simulink model "DigitalTwin_AI"  (R2024b)
settings: Solver=FixedStepAuto  StartTime=0.0  StopTime=60  FixedStep=0.05  RelTol=1e-3
libraries: dspadpt3 x1
settings Model: Creator=dossantos  LastModifiedBy=dossantos

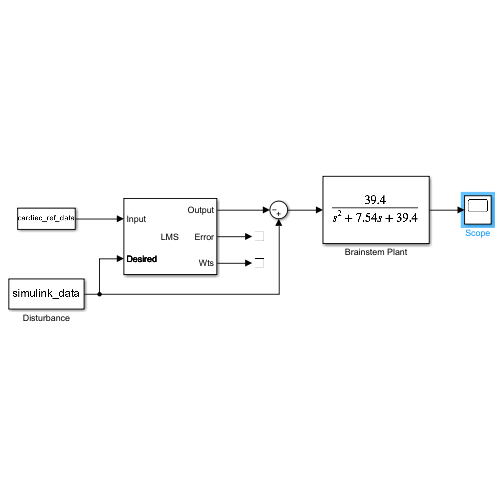
[thumbnail: Simulink's stored preview of the top-level diagram]
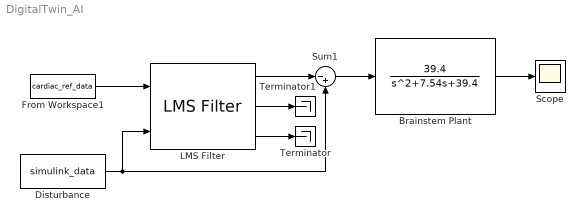
== system DigitalTwin_AI ==
  Brainstem Plant : TransferFcn  Numerator=[39.4]  Denominator=[1 7.54 39.4]
  Disturbance : FromWorkspace  VariableName=simulink_data  SampleTime=0.05  Interpolate=off  OutputAfterFinalValue=Cyclic repetition
  From Workspace1 : FromWorkspace  VariableName=cardiac_ref_data  SampleTime=0.05  Interpolate=off  OutputAfterFinalValue=Cyclic repetition
  LMS Filter : dspadpt3/LMS Filter  Algo=LMS  L=32  stepflag=Dialog  mu=0.01  leakage=1.0  ic=0  Adapt=off  resetflag=None  weights=on  addnparflag=off  roundingMode=Floor  overflowMode=off
  Scope : Scope
  Sum1 : Sum  Inputs=|-+
  Terminator : Terminator
  Terminator1 : Terminator
  wires:
  Brainstem Plant/1 -> Scope/1
  Sum1/1 -> Brainstem Plant/1
  Disturbance/1 -> LMS Filter/2, Sum1/2
  From Workspace1/1 -> LMS Filter/1
  LMS Filter/3 -> Terminator/1
  LMS Filter/2 -> Terminator1/1
  LMS Filter/1 -> Sum1/1
